simulink model "Ejercicio2Difuso"  (R2025a)
settings: Solver=VariableStepAuto  StartTime=0.0  StopTime=10.0  MaxStep=1e-2  RelTol=1e-3
settings Model: Creator=user  LastModifiedBy=Estudiantes

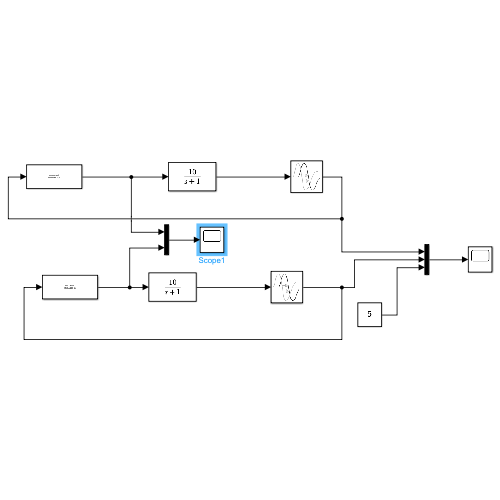
[thumbnail: Simulink's stored preview of the top-level diagram]
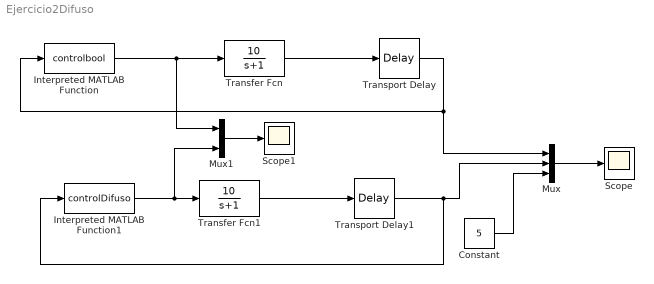
== system Ejercicio2Difuso ==
  Constant : Constant  Value=5
  Interpreted MATLAB Function : MATLABFcn  MATLABFcn=controlbool
  Interpreted MATLAB Function1 : MATLABFcn  MATLABFcn=controlDifuso
  Mux : Mux  Inputs=3
  Mux1 : Mux  Inputs=2
  Scope : Scope
      settings: ActiveDisplayYMinimum=-6.2903518392080535  ActiveDisplayYMaximum=15.899685158419963
  Scope1 : Scope
      settings: ActiveDisplayYMinimum=-0.37499999999999989  ActiveDisplayYMaximum=3.375
  Transfer Fcn : TransferFcn  Numerator=[10]  Denominator=[1 1]
  Transfer Fcn1 : TransferFcn  Numerator=[10]  Denominator=[1 1]
  Transport Delay : TransportDelay  DelayTime=0.5
  Transport Delay1 : TransportDelay  DelayTime=0.5
  wires:
  Interpreted MATLAB Function/1 -> Mux1/1, Transfer Fcn/1
  Transfer Fcn/1 -> Transport Delay/1
  Transport Delay/1 -> Mux/1, Interpreted MATLAB Function/1
  Transfer Fcn1/1 -> Transport Delay1/1
  Interpreted MATLAB Function1/1 -> Mux1/2, Transfer Fcn1/1
  Mux/1 -> Scope/1
  Transport Delay1/1 -> Interpreted MATLAB Function1/1, Mux/2
  Constant/1 -> Mux/3
  Mux1/1 -> Scope1/1
